simulink model "week1problem9"  (R2020b)
settings: Solver=VariableStepAuto  StartTime=0.0  StopTime=10.0  RelTol=1e-3
model workspace (MAT data in the model file):
  Ki = 1
  L = Simulink.Parameter
  L.Value = 1
  L.DataType = 'auto'
  L.Dimensions = [1 1]
  R = Simulink.Parameter
  R.Value = 1.2
  R.DataType = 'auto'
  R.Dimensions = [1 1]
settings Model: Creator=HP  LastModifiedBy=HP

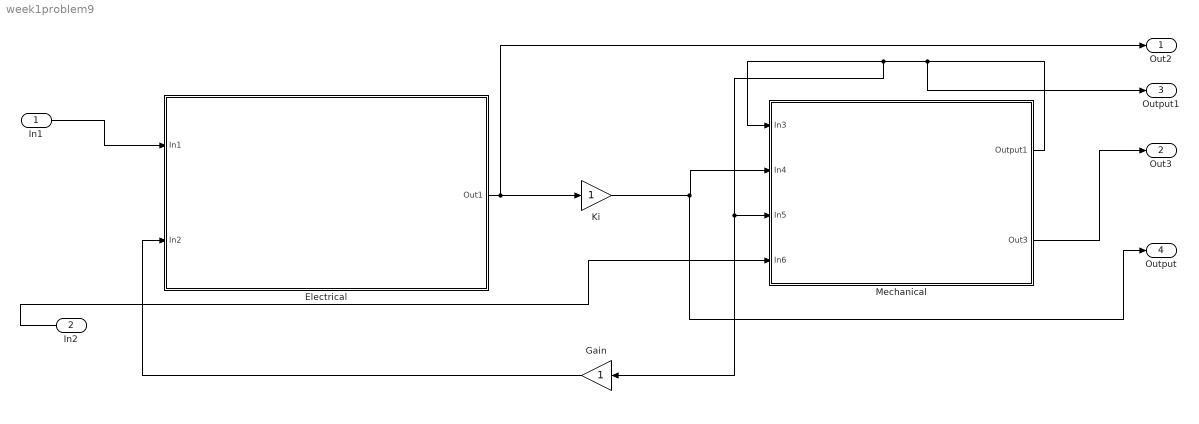
== system week1problem9 ==
  In1 : Inport
  In2 : Inport  Port=2
  Electrical : Subsystem
  Gain : Gain
  Ki : Gain
  Mechanical : Subsystem
  Out2 : Outport
  Out3 : Outport  Port=2
  Output1 : Outport  Port=3
  Output : Outport  Port=4
  wires:
  In1/1 -> Electrical/1(In1)
  Mechanical/2(Out3) -> Out3/1
  Gain/1 -> Electrical/2(In2)
  Electrical/1(Out1) -> Out2/1, Ki/1
  Mechanical/1(Output1) -> Output1/1, Mechanical/3(In5), Gain/1, Mechanical/1(In3)
  Ki/1 -> Output/1, Mechanical/2(In4)
  In2/1 -> Mechanical/4(In6)

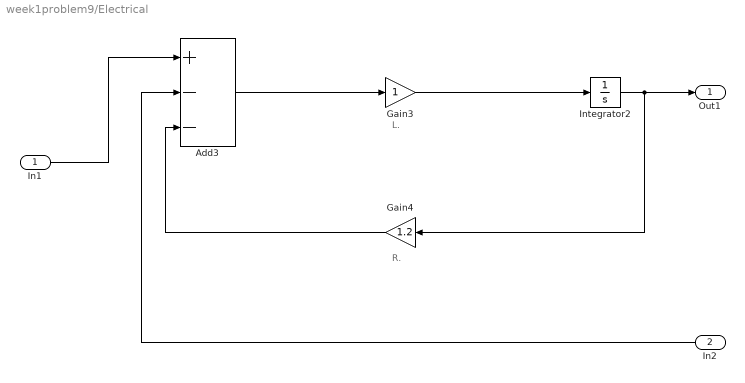
== system week1problem9/Electrical ==
  note: L.
  note: R.
  In1 : Inport
  In2 : Inport  Port=2
  Add3 : Sum  Inputs=+--
  Gain3 : Gain
  Gain4 : Gain  Gain=1.2
  Integrator2 : Integrator
  Out1 : Outport
  wires:
  Gain4/1 -> Add3/3
  In2/1 -> Add3/2
  Integrator2/1 -> Out1/1, Gain4/1
  In1/1 -> Add3/1
  Add3/1 -> Gain3/1
  Gain3/1 -> Integrator2/1

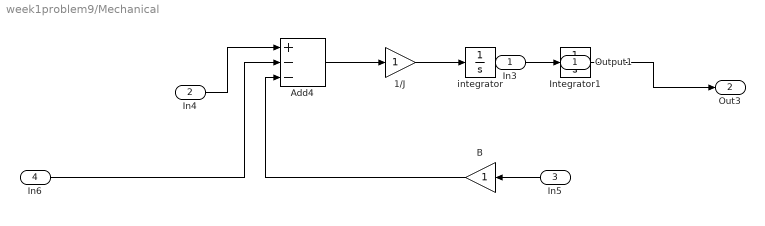
== system week1problem9/Mechanical ==
  In3 : Inport
  In4 : Inport  Port=2
  In5 : Inport  Port=3
  In6 : Inport  Port=4
  1/J : Gain
  Add4 : Sum  Inputs=+--
  B : Gain
  Integrator1 : Integrator
  integrator : Integrator
  Output1 : Outport
  Out3 : Outport  Port=2
  wires:
  In6/1 -> Add4/2
  In3/1 -> Integrator1/1
  1/J/1 -> integrator/1
  B/1 -> Add4/3
  Integrator1/1 -> Out3/1
  In5/1 -> B/1
  In4/1 -> Add4/1
  Add4/1 -> 1/J/1
  integrator/1 -> Output1/1
